simulink model "ScriptDemo"  (R2022b)
settings: configuration reference "TmVcThermal_Configuration_sub" (kept outside this file)
undefined symbols (not defined in the file or in its folder): aaaa, bbbb, cTmComprCtrl_D_u8HvacFlowTable_db, cTmComprCtrl_D_u8HvacFlowTable_sw, cTmComprCtrl_n_i16ChillCmpIMax, cTmComprCtrl_n_i16ChillCmpIMin, cTmComprCtrl_n_i16ChillCmpIMin666, cTmComprCtrl_n_i16ChillCmpPMax, cTmComprCtrl_n_i16ChillCmpPMin, cTmComprCtrl_n_i16CmpChillCoolRpmKiMax, cTmComprCtrl_n_i16CmpChillCoolRpmKiMin, cTmComprCtrl_n_i16CmpChillCoolRpmKpMax, cTmComprCtrl_n_i16CmpChillCoolRpmKpMin, cTmComprCtrl_n_i16CmpCoolRpmKiMax, cTmComprCtrl_n_i16CmpCoolRpmKiMin, cTmComprCtrl_n_i16CmpCoolRpmKpMax, cTmComprCtrl_n_i16CmpCoolRpmKpMin, cTmComprCtrl_n_i16SM4CmpHeatKiMax, cTmComprCtrl_n_i16SM4CmpHeatKiMin, cTmComprCtrl_n_i16SM4CmpHeatKpMax, cTmComprCtrl_n_i16SM4CmpHeatKpMin, cTmComprCtrl_n_i16SM5CmpHeatKiMax, cTmComprCtrl_n_i16SM5CmpHeatKiMin, cTmComprCtrl_n_i16SM5CmpHeatKpMax, cTmComprCtrl_n_i16SM5CmpHeatKpMin, cTmComprCtrl_n_i16SM6CmpHeatKiMax, cTmComprCtrl_n_i16SM6CmpHeatKiMin, cTmComprCtrl_n_i16SM6CmpHeatKpMax, cTmComprCtrl_n_i16SM6CmpHeatKpMin, cTmComprCtrl_n_u16CmpMaxSpdFanFltLimt, cTmComprCtrl_n_u16CmpMaxSpdLoSidePFltLimt, cTmComprCtrl_n_u16CmpMaxSpdSensorFltLimt, cTmComprCtrl_n_u16CompMinRpm, cTmComprCtrl_n_u16CompRpmIncThres, cTmComprCtrl_t_u16BattCooltFFPeriod, cTmComprCtrl_t_u16BattCooltPIPeriod, cTmComprCtrl_t_u16CmpCoolFFPeriod, cTmComprCtrl_t_u16CmpCoolPIPeriod, cTmComprCtrl_t_u16CoolCmpChillFFPeriod, cTmComprCtrl_t_u16CoolCmpChillPIPeriod, cTmComprCtrl_t_u16SM4CmpHeatFFPeriod, cTmComprCtrl_t_u16SM4CmpHeatPIPeriod, cTmComprCtrl_t_u16SM5CmpHeatFFPeriod, cTmComprCtrl_t_u16SM5CmpHeatPIPeriod, cTmComprCtrl_t_u16SM6CmpHeatFFPeriod, cTmComprCtrl_t_u16SM6CmpHeatPIPeriod, cTmComprCtrl_Te_EvapClearInteg, cTmComprCtrl_Te_i16HpReqTempSaturoffset, cTmComprCtrl_Te_i16SatLpReplaceDiff, cTmComprCtrl_Te_i16SM3BatDiffStartEvapDecOffset, cTmComprCtrl_Te_i16SM3EvapLo, cTmComprCtrl_Te_i16SM3TBatDiffEntEvapDecOffset, cTmComprCtrl_Te_i16SM3TBatDiffEntEvapDecOffsetQuit, cTmComprCtrl_Te_s32ErrCmpChillPIContinueCoolH, cTmComprCtrl_Te_s32ErrCmpChillPIContinueCoolL, cTmComprCtrl_Te_s32ErrCmpPIContinueChillH, cTmComprCtrl_Te_s32ErrCmpPIContinueChillL, cTmComprCtrl_Te_s32ErrCmpPIContinueCoolH, cTmComprCtrl_Te_s32ErrCmpPIContinueCoolL, cTmComprCtrl_Te_s32ErrCmpPIContinueHeatH ... (+398)
libraries: simulink x846, PCMULib x711, simulink_need_slupdate x4
(part 11 of 49)

== system ScriptDemo/Create/createSigOnLine/After ==
  note: createSigOnLine(gcs ,'resoveValue',true)
  sTmRefriVlvCtrl_X_s32CEXVPosReqIn : Inport  OutDataTypeStr=single  OutputFunctionCall=on
  sTmRefriVlvCtrl_X_s32EEXVPosReqIn : Inport  Port=2  OutDataTypeStr=single
  sTmRefriVlvCtrl_X_s32BEXVPosReqIn : Inport  Port=3  OutDataTypeStr=single
  yTmRefriVlvCtrl_B_HpcCexvMovEnableIn : Inport  Port=4  OutDataTypeStr=boolean
  sTmRefriVlvCtrl_Z_u8CEXVInitStateIn : Inport  Port=5  OutDataTypeStr=uint8
  yTmRefriVlvCtrl_B_CexvCalibReqIn : Inport  Port=6  OutDataTypeStr=boolean
  yTmRefriVlvCtrl_B_HpcEexvMovEnableIn : Inport  Port=7  OutDataTypeStr=boolean
  sTmRefriVlvCtrl_Z_u8EEXVInitStateIn : Inport  Port=8  OutDataTypeStr=uint8
  yTmRefriVlvCtrl_B_EexvCalibReqIn : Inport  Port=9  OutDataTypeStr=boolean
  yTmRefriVlvCtrl_B_HpcBexvMovEnableIn : Inport  Port=10  OutDataTypeStr=boolean
  sTmRefriVlvCtrl_Z_u8BEXVInitStateIn : Inport  Port=11  OutDataTypeStr=uint8
  yTmRefriVlvCtrl_B_BexvCalibReqIn : Inport  Port=12  OutDataTypeStr=boolean
  sTmRefriVlvCtrl_X_s32SM3BexvMaxPosIn : Inport  Port=13  OutDataTypeStr=single
  yTmRefriVlvCtrl_B_EvapBattTLimBexvEnaIn : Inport  Port=14  OutDataTypeStr=boolean
  sTmRefriVlvCtrl_D_u8EexvRefriSwitchStIn : Inport  Port=15  OutDataTypeStr=uint8
  sTmRefriVlvCtrl_D_u8CexvRefriSwitchStIn : Inport  Port=16  OutDataTypeStr=uint8
  sTmRefriVlvCtrl_D_u8BexvRefriSwitchStIn : Inport  Port=17  OutDataTypeStr=uint8
  Before : Subsystem
  sTmRefriVlvCtrl_X_s32CEXVPosReq : Outport  OutDataTypeStr=single
  sTmRefriVlvCtrl_X_s32EEXVPosReq : Outport  Port=2  OutDataTypeStr=single
  sTmRefriVlvCtrl_X_s32BEXVPosReq : Outport  Port=3  OutDataTypeStr=single
  yTmRefriVlvCtrl_B_HpcCexvMovEnable : Outport  Port=4  OutDataTypeStr=boolean
  sTmRefriVlvCtrl_Z_u8CEXVInitState : Outport  Port=5  OutDataTypeStr=uint8
  yTmRefriVlvCtrl_B_CexvCalibReq : Outport  Port=6  OutDataTypeStr=boolean
  yTmRefriVlvCtrl_B_HpcEexvMovEnable : Outport  Port=7  OutDataTypeStr=boolean
  sTmRefriVlvCtrl_Z_u8EEXVInitState : Outport  Port=8  OutDataTypeStr=uint8
  yTmRefriVlvCtrl_B_EexvCalibReq : Outport  Port=9  OutDataTypeStr=boolean
  yTmRefriVlvCtrl_B_HpcBexvMovEnable : Outport  Port=10  OutDataTypeStr=boolean
  sTmRefriVlvCtrl_Z_u8BEXVInitState : Outport  Port=11  OutDataTypeStr=uint8
  yTmRefriVlvCtrl_B_BexvCalibReq : Outport  Port=12  OutDataTypeStr=boolean
  sTmRefriVlvCtrl_X_s32SM3BexvMaxPos : Outport  Port=13  OutDataTypeStr=single
  yTmRefriVlvCtrl_B_EvapBattTLimBexvEna : Outport  Port=14  OutDataTypeStr=boolean
  sTmRefriVlvCtrl_D_u8EexvRefriSwitchSt : Outport  Port=15  OutDataTypeStr=uint8
  sTmRefriVlvCtrl_D_u8CexvRefriSwitchSt : Outport  Port=16  OutDataTypeStr=uint8
  sTmRefriVlvCtrl_D_u8BexvRefriSwitchSt : Outport  Port=17  OutDataTypeStr=uint8
  wires:
  Before/17(sTmRefriVlvCtrl_D_u8BexvRefriSwitchSt) -> sTmRefriVlvCtrl_D_u8BexvRefriSwitchSt/1  "sTmRefriVlvCtrl_D_u8BexvRefriSwitchSt"
  Before/3(sTmRefriVlvCtrl_X_s32BEXVPosReq) -> sTmRefriVlvCtrl_X_s32BEXVPosReq/1  "sTmRefriVlvCtrl_X_s32BEXVPosReq"
  Before/11(sTmRefriVlvCtrl_Z_u8BEXVInitState) -> sTmRefriVlvCtrl_Z_u8BEXVInitState/1  "sTmRefriVlvCtrl_Z_u8BEXVInitState"
  Before/10(yTmRefriVlvCtrl_B_HpcBexvMovEnable) -> yTmRefriVlvCtrl_B_HpcBexvMovEnable/1  "yTmRefriVlvCtrl_B_HpcBexvMovEnable"
  Before/15(sTmRefriVlvCtrl_D_u8EexvRefriSwitchSt) -> sTmRefriVlvCtrl_D_u8EexvRefriSwitchSt/1  "sTmRefriVlvCtrl_D_u8EexvRefriSwitchSt"
  Before/7(yTmRefriVlvCtrl_B_HpcEexvMovEnable) -> yTmRefriVlvCtrl_B_HpcEexvMovEnable/1  "yTmRefriVlvCtrl_B_HpcEexvMovEnable"
  Before/14(yTmRefriVlvCtrl_B_EvapBattTLimBexvEna) -> yTmRefriVlvCtrl_B_EvapBattTLimBexvEna/1  "yTmRefriVlvCtrl_B_EvapBattTLimBexvEna"
  Before/12(yTmRefriVlvCtrl_B_BexvCalibReq) -> yTmRefriVlvCtrl_B_BexvCalibReq/1  "yTmRefriVlvCtrl_B_BexvCalibReq"
  Before/9(yTmRefriVlvCtrl_B_EexvCalibReq) -> yTmRefriVlvCtrl_B_EexvCalibReq/1  "yTmRefriVlvCtrl_B_EexvCalibReq"
  Before/5(sTmRefriVlvCtrl_Z_u8CEXVInitState) -> sTmRefriVlvCtrl_Z_u8CEXVInitState/1  "sTmRefriVlvCtrl_Z_u8CEXVInitState"
  Before/13(sTmRefriVlvCtrl_X_s32SM3BexvMaxPos) -> sTmRefriVlvCtrl_X_s32SM3BexvMaxPos/1  "sTmRefriVlvCtrl_X_s32SM3BexvMaxPos"
  Before/4(yTmRefriVlvCtrl_B_HpcCexvMovEnable) -> yTmRefriVlvCtrl_B_HpcCexvMovEnable/1  "yTmRefriVlvCtrl_B_HpcCexvMovEnable"
  sTmRefriVlvCtrl_D_u8EexvRefriSwitchStIn/1 -> Before/15(sTmRefriVlvCtrl_D_u8EexvRefriSwitchStIn)  "sTmRefriVlvCtrl_D_u8EexvRefriSwitchStIn"
  yTmRefriVlvCtrl_B_CexvCalibReqIn/1 -> Before/6(yTmRefriVlvCtrl_B_CexvCalibReqIn)  "yTmRefriVlvCtrl_B_CexvCalibReqIn"
  sTmRefriVlvCtrl_D_u8BexvRefriSwitchStIn/1 -> Before/17(sTmRefriVlvCtrl_D_u8BexvRefriSwitchStIn)  "sTmRefriVlvCtrl_D_u8BexvRefriSwitchStIn"
  Before/16(sTmRefriVlvCtrl_D_u8CexvRefriSwitchSt) -> sTmRefriVlvCtrl_D_u8CexvRefriSwitchSt/1  "sTmRefriVlvCtrl_D_u8CexvRefriSwitchSt"
  Before/2(sTmRefriVlvCtrl_X_s32EEXVPosReq) -> sTmRefriVlvCtrl_X_s32EEXVPosReq/1  "sTmRefriVlvCtrl_X_s32EEXVPosReq"
  sTmRefriVlvCtrl_D_u8CexvRefriSwitchStIn/1 -> Before/16(sTmRefriVlvCtrl_D_u8CexvRefriSwitchStIn)  "sTmRefriVlvCtrl_D_u8CexvRefriSwitchStIn"
  yTmRefriVlvCtrl_B_HpcCexvMovEnableIn/1 -> Before/4(yTmRefriVlvCtrl_B_HpcCexvMovEnableIn)  "yTmRefriVlvCtrl_B_HpcCexvMovEnableIn"
  yTmRefriVlvCtrl_B_BexvCalibReqIn/1 -> Before/12(yTmRefriVlvCtrl_B_BexvCalibReqIn)  "yTmRefriVlvCtrl_B_BexvCalibReqIn"
  Before/6(yTmRefriVlvCtrl_B_CexvCalibReq) -> yTmRefriVlvCtrl_B_CexvCalibReq/1  "yTmRefriVlvCtrl_B_CexvCalibReq"
  sTmRefriVlvCtrl_X_s32SM3BexvMaxPosIn/1 -> Before/13(sTmRefriVlvCtrl_X_s32SM3BexvMaxPosIn)  "sTmRefriVlvCtrl_X_s32SM3BexvMaxPosIn"
  yTmRefriVlvCtrl_B_HpcEexvMovEnableIn/1 -> Before/7(yTmRefriVlvCtrl_B_HpcEexvMovEnableIn)  "yTmRefriVlvCtrl_B_HpcEexvMovEnableIn"
  yTmRefriVlvCtrl_B_EexvCalibReqIn/1 -> Before/9(yTmRefriVlvCtrl_B_EexvCalibReqIn)  "yTmRefriVlvCtrl_B_EexvCalibReqIn"
  sTmRefriVlvCtrl_Z_u8CEXVInitStateIn/1 -> Before/5(sTmRefriVlvCtrl_Z_u8CEXVInitStateIn)  "sTmRefriVlvCtrl_Z_u8CEXVInitStateIn"
  sTmRefriVlvCtrl_Z_u8BEXVInitStateIn/1 -> Before/11(sTmRefriVlvCtrl_Z_u8BEXVInitStateIn)  "sTmRefriVlvCtrl_Z_u8BEXVInitStateIn"
  sTmRefriVlvCtrl_X_s32BEXVPosReqIn/1 -> Before/3(sTmRefriVlvCtrl_X_s32BEXVPosReqIn)  "sTmRefriVlvCtrl_X_s32BEXVPosReqIn"
  Before/1(sTmRefriVlvCtrl_X_s32CEXVPosReq) -> sTmRefriVlvCtrl_X_s32CEXVPosReq/1  "sTmRefriVlvCtrl_X_s32CEXVPosReq"
  yTmRefriVlvCtrl_B_HpcBexvMovEnableIn/1 -> Before/10(yTmRefriVlvCtrl_B_HpcBexvMovEnableIn)  "yTmRefriVlvCtrl_B_HpcBexvMovEnableIn"
  sTmRefriVlvCtrl_X_s32EEXVPosReqIn/1 -> Before/2(sTmRefriVlvCtrl_X_s32EEXVPosReqIn)  "sTmRefriVlvCtrl_X_s32EEXVPosReqIn"
  sTmRefriVlvCtrl_Z_u8EEXVInitStateIn/1 -> Before/8(sTmRefriVlvCtrl_Z_u8EEXVInitStateIn)  "sTmRefriVlvCtrl_Z_u8EEXVInitStateIn"
  Before/8(sTmRefriVlvCtrl_Z_u8EEXVInitState) -> sTmRefriVlvCtrl_Z_u8EEXVInitState/1  "sTmRefriVlvCtrl_Z_u8EEXVInitState"
  sTmRefriVlvCtrl_X_s32CEXVPosReqIn/1 -> Before/1(sTmRefriVlvCtrl_X_s32CEXVPosReqIn)  "sTmRefriVlvCtrl_X_s32CEXVPosReqIn"
  yTmRefriVlvCtrl_B_EvapBattTLimBexvEnaIn/1 -> Before/14(yTmRefriVlvCtrl_B_EvapBattTLimBexvEnaIn)  "yTmRefriVlvCtrl_B_EvapBattTLimBexvEnaIn"

== system ScriptDemo/Create/createSigOnLine/After2 ==
  note: createSigOnLine(gcs ,'logValue',true)
  sTmRefriVlvCtrl_X_s32CEXVPosReqIn : Inport  OutDataTypeStr=single  OutputFunctionCall=on
  sTmRefriVlvCtrl_X_s32EEXVPosReqIn : Inport  Port=2  OutDataTypeStr=single
  sTmRefriVlvCtrl_X_s32BEXVPosReqIn : Inport  Port=3  OutDataTypeStr=single
  yTmRefriVlvCtrl_B_HpcCexvMovEnableIn : Inport  Port=4  OutDataTypeStr=boolean
  sTmRefriVlvCtrl_Z_u8CEXVInitStateIn : Inport  Port=5  OutDataTypeStr=uint8
  yTmRefriVlvCtrl_B_CexvCalibReqIn : Inport  Port=6  OutDataTypeStr=boolean
  yTmRefriVlvCtrl_B_HpcEexvMovEnableIn : Inport  Port=7  OutDataTypeStr=boolean
  sTmRefriVlvCtrl_Z_u8EEXVInitStateIn : Inport  Port=8  OutDataTypeStr=uint8
  yTmRefriVlvCtrl_B_EexvCalibReqIn : Inport  Port=9  OutDataTypeStr=boolean
  yTmRefriVlvCtrl_B_HpcBexvMovEnableIn : Inport  Port=10  OutDataTypeStr=boolean
  sTmRefriVlvCtrl_Z_u8BEXVInitStateIn : Inport  Port=11  OutDataTypeStr=uint8
  yTmRefriVlvCtrl_B_BexvCalibReqIn : Inport  Port=12  OutDataTypeStr=boolean
  sTmRefriVlvCtrl_X_s32SM3BexvMaxPosIn : Inport  Port=13  OutDataTypeStr=single
  yTmRefriVlvCtrl_B_EvapBattTLimBexvEnaIn : Inport  Port=14  OutDataTypeStr=boolean
  sTmRefriVlvCtrl_D_u8EexvRefriSwitchStIn : Inport  Port=15  OutDataTypeStr=uint8
  sTmRefriVlvCtrl_D_u8CexvRefriSwitchStIn : Inport  Port=16  OutDataTypeStr=uint8
  sTmRefriVlvCtrl_D_u8BexvRefriSwitchStIn : Inport  Port=17  OutDataTypeStr=uint8
  Before : Subsystem
  sTmRefriVlvCtrl_X_s32CEXVPosReq : Outport  OutDataTypeStr=single
  sTmRefriVlvCtrl_X_s32EEXVPosReq : Outport  Port=2  OutDataTypeStr=single
  sTmRefriVlvCtrl_X_s32BEXVPosReq : Outport  Port=3  OutDataTypeStr=single
  yTmRefriVlvCtrl_B_HpcCexvMovEnable : Outport  Port=4  OutDataTypeStr=boolean
  sTmRefriVlvCtrl_Z_u8CEXVInitState : Outport  Port=5  OutDataTypeStr=uint8
  yTmRefriVlvCtrl_B_CexvCalibReq : Outport  Port=6  OutDataTypeStr=boolean
  yTmRefriVlvCtrl_B_HpcEexvMovEnable : Outport  Port=7  OutDataTypeStr=boolean
  sTmRefriVlvCtrl_Z_u8EEXVInitState : Outport  Port=8  OutDataTypeStr=uint8
  yTmRefriVlvCtrl_B_EexvCalibReq : Outport  Port=9  OutDataTypeStr=boolean
  yTmRefriVlvCtrl_B_HpcBexvMovEnable : Outport  Port=10  OutDataTypeStr=boolean
  sTmRefriVlvCtrl_Z_u8BEXVInitState : Outport  Port=11  OutDataTypeStr=uint8
  yTmRefriVlvCtrl_B_BexvCalibReq : Outport  Port=12  OutDataTypeStr=boolean
  sTmRefriVlvCtrl_X_s32SM3BexvMaxPos : Outport  Port=13  OutDataTypeStr=single
  yTmRefriVlvCtrl_B_EvapBattTLimBexvEna : Outport  Port=14  OutDataTypeStr=boolean
  sTmRefriVlvCtrl_D_u8EexvRefriSwitchSt : Outport  Port=15  OutDataTypeStr=uint8
  sTmRefriVlvCtrl_D_u8CexvRefriSwitchSt : Outport  Port=16  OutDataTypeStr=uint8
  sTmRefriVlvCtrl_D_u8BexvRefriSwitchSt : Outport  Port=17  OutDataTypeStr=uint8
  wires:
  Before/17(sTmRefriVlvCtrl_D_u8BexvRefriSwitchSt) -> sTmRefriVlvCtrl_D_u8BexvRefriSwitchSt/1  "sTmRefriVlvCtrl_D_u8BexvRefriSwitchSt"
  Before/3(sTmRefriVlvCtrl_X_s32BEXVPosReq) -> sTmRefriVlvCtrl_X_s32BEXVPosReq/1  "sTmRefriVlvCtrl_X_s32BEXVPosReq"
  Before/11(sTmRefriVlvCtrl_Z_u8BEXVInitState) -> sTmRefriVlvCtrl_Z_u8BEXVInitState/1  "sTmRefriVlvCtrl_Z_u8BEXVInitState"
  Before/10(yTmRefriVlvCtrl_B_HpcBexvMovEnable) -> yTmRefriVlvCtrl_B_HpcBexvMovEnable/1  "yTmRefriVlvCtrl_B_HpcBexvMovEnable"
  Before/15(sTmRefriVlvCtrl_D_u8EexvRefriSwitchSt) -> sTmRefriVlvCtrl_D_u8EexvRefriSwitchSt/1  "sTmRefriVlvCtrl_D_u8EexvRefriSwitchSt"
  Before/7(yTmRefriVlvCtrl_B_HpcEexvMovEnable) -> yTmRefriVlvCtrl_B_HpcEexvMovEnable/1  "yTmRefriVlvCtrl_B_HpcEexvMovEnable"
  Before/14(yTmRefriVlvCtrl_B_EvapBattTLimBexvEna) -> yTmRefriVlvCtrl_B_EvapBattTLimBexvEna/1  "yTmRefriVlvCtrl_B_EvapBattTLimBexvEna"
  Before/12(yTmRefriVlvCtrl_B_BexvCalibReq) -> yTmRefriVlvCtrl_B_BexvCalibReq/1  "yTmRefriVlvCtrl_B_BexvCalibReq"
  Before/9(yTmRefriVlvCtrl_B_EexvCalibReq) -> yTmRefriVlvCtrl_B_EexvCalibReq/1  "yTmRefriVlvCtrl_B_EexvCalibReq"
  Before/5(sTmRefriVlvCtrl_Z_u8CEXVInitState) -> sTmRefriVlvCtrl_Z_u8CEXVInitState/1  "sTmRefriVlvCtrl_Z_u8CEXVInitState"
  Before/13(sTmRefriVlvCtrl_X_s32SM3BexvMaxPos) -> sTmRefriVlvCtrl_X_s32SM3BexvMaxPos/1  "sTmRefriVlvCtrl_X_s32SM3BexvMaxPos"
  Before/4(yTmRefriVlvCtrl_B_HpcCexvMovEnable) -> yTmRefriVlvCtrl_B_HpcCexvMovEnable/1  "yTmRefriVlvCtrl_B_HpcCexvMovEnable"
  sTmRefriVlvCtrl_D_u8EexvRefriSwitchStIn/1 -> Before/15(sTmRefriVlvCtrl_D_u8EexvRefriSwitchStIn)  "sTmRefriVlvCtrl_D_u8EexvRefriSwitchStIn"
  yTmRefriVlvCtrl_B_CexvCalibReqIn/1 -> Before/6(yTmRefriVlvCtrl_B_CexvCalibReqIn)  "yTmRefriVlvCtrl_B_CexvCalibReqIn"
  sTmRefriVlvCtrl_D_u8BexvRefriSwitchStIn/1 -> Before/17(sTmRefriVlvCtrl_D_u8BexvRefriSwitchStIn)  "sTmRefriVlvCtrl_D_u8BexvRefriSwitchStIn"
  Before/16(sTmRefriVlvCtrl_D_u8CexvRefriSwitchSt) -> sTmRefriVlvCtrl_D_u8CexvRefriSwitchSt/1  "sTmRefriVlvCtrl_D_u8CexvRefriSwitchSt"
  Before/2(sTmRefriVlvCtrl_X_s32EEXVPosReq) -> sTmRefriVlvCtrl_X_s32EEXVPosReq/1  "sTmRefriVlvCtrl_X_s32EEXVPosReq"
  sTmRefriVlvCtrl_D_u8CexvRefriSwitchStIn/1 -> Before/16(sTmRefriVlvCtrl_D_u8CexvRefriSwitchStIn)  "sTmRefriVlvCtrl_D_u8CexvRefriSwitchStIn"
  yTmRefriVlvCtrl_B_HpcCexvMovEnableIn/1 -> Before/4(yTmRefriVlvCtrl_B_HpcCexvMovEnableIn)  "yTmRefriVlvCtrl_B_HpcCexvMovEnableIn"
  yTmRefriVlvCtrl_B_BexvCalibReqIn/1 -> Before/12(yTmRefriVlvCtrl_B_BexvCalibReqIn)  "yTmRefriVlvCtrl_B_BexvCalibReqIn"
  Before/6(yTmRefriVlvCtrl_B_CexvCalibReq) -> yTmRefriVlvCtrl_B_CexvCalibReq/1  "yTmRefriVlvCtrl_B_CexvCalibReq"
  sTmRefriVlvCtrl_X_s32SM3BexvMaxPosIn/1 -> Before/13(sTmRefriVlvCtrl_X_s32SM3BexvMaxPosIn)  "sTmRefriVlvCtrl_X_s32SM3BexvMaxPosIn"
  yTmRefriVlvCtrl_B_HpcEexvMovEnableIn/1 -> Before/7(yTmRefriVlvCtrl_B_HpcEexvMovEnableIn)  "yTmRefriVlvCtrl_B_HpcEexvMovEnableIn"
  yTmRefriVlvCtrl_B_EexvCalibReqIn/1 -> Before/9(yTmRefriVlvCtrl_B_EexvCalibReqIn)  "yTmRefriVlvCtrl_B_EexvCalibReqIn"
  sTmRefriVlvCtrl_Z_u8CEXVInitStateIn/1 -> Before/5(sTmRefriVlvCtrl_Z_u8CEXVInitStateIn)  "sTmRefriVlvCtrl_Z_u8CEXVInitStateIn"
  sTmRefriVlvCtrl_Z_u8BEXVInitStateIn/1 -> Before/11(sTmRefriVlvCtrl_Z_u8BEXVInitStateIn)  "sTmRefriVlvCtrl_Z_u8BEXVInitStateIn"
  sTmRefriVlvCtrl_X_s32BEXVPosReqIn/1 -> Before/3(sTmRefriVlvCtrl_X_s32BEXVPosReqIn)  "sTmRefriVlvCtrl_X_s32BEXVPosReqIn"
  Before/1(sTmRefriVlvCtrl_X_s32CEXVPosReq) -> sTmRefriVlvCtrl_X_s32CEXVPosReq/1  "sTmRefriVlvCtrl_X_s32CEXVPosReq"
  yTmRefriVlvCtrl_B_HpcBexvMovEnableIn/1 -> Before/10(yTmRefriVlvCtrl_B_HpcBexvMovEnableIn)  "yTmRefriVlvCtrl_B_HpcBexvMovEnableIn"
  sTmRefriVlvCtrl_X_s32EEXVPosReqIn/1 -> Before/2(sTmRefriVlvCtrl_X_s32EEXVPosReqIn)  "sTmRefriVlvCtrl_X_s32EEXVPosReqIn"
  sTmRefriVlvCtrl_Z_u8EEXVInitStateIn/1 -> Before/8(sTmRefriVlvCtrl_Z_u8EEXVInitStateIn)  "sTmRefriVlvCtrl_Z_u8EEXVInitStateIn"
  Before/8(sTmRefriVlvCtrl_Z_u8EEXVInitState) -> sTmRefriVlvCtrl_Z_u8EEXVInitState/1  "sTmRefriVlvCtrl_Z_u8EEXVInitState"
  sTmRefriVlvCtrl_X_s32CEXVPosReqIn/1 -> Before/1(sTmRefriVlvCtrl_X_s32CEXVPosReqIn)  "sTmRefriVlvCtrl_X_s32CEXVPosReqIn"
  yTmRefriVlvCtrl_B_EvapBattTLimBexvEnaIn/1 -> Before/14(yTmRefriVlvCtrl_B_EvapBattTLimBexvEnaIn)  "yTmRefriVlvCtrl_B_EvapBattTLimBexvEnaIn"

== system ScriptDemo/Create/createSigOnLine/After3 ==
  note: createSigOnLine(gcs ,' testValue ',true)
  sTmRefriVlvCtrl_X_s32CEXVPosReqIn : Inport  OutDataTypeStr=single  OutputFunctionCall=on
  sTmRefriVlvCtrl_X_s32EEXVPosReqIn : Inport  Port=2  OutDataTypeStr=single
  sTmRefriVlvCtrl_X_s32BEXVPosReqIn : Inport  Port=3  OutDataTypeStr=single
  yTmRefriVlvCtrl_B_HpcCexvMovEnableIn : Inport  Port=4  OutDataTypeStr=boolean
  sTmRefriVlvCtrl_Z_u8CEXVInitStateIn : Inport  Port=5  OutDataTypeStr=uint8
  yTmRefriVlvCtrl_B_CexvCalibReqIn : Inport  Port=6  OutDataTypeStr=boolean
  yTmRefriVlvCtrl_B_HpcEexvMovEnableIn : Inport  Port=7  OutDataTypeStr=boolean
  sTmRefriVlvCtrl_Z_u8EEXVInitStateIn : Inport  Port=8  OutDataTypeStr=uint8
  yTmRefriVlvCtrl_B_EexvCalibReqIn : Inport  Port=9  OutDataTypeStr=boolean
  yTmRefriVlvCtrl_B_HpcBexvMovEnableIn : Inport  Port=10  OutDataTypeStr=boolean
  sTmRefriVlvCtrl_Z_u8BEXVInitStateIn : Inport  Port=11  OutDataTypeStr=uint8
  yTmRefriVlvCtrl_B_BexvCalibReqIn : Inport  Port=12  OutDataTypeStr=boolean
  sTmRefriVlvCtrl_X_s32SM3BexvMaxPosIn : Inport  Port=13  OutDataTypeStr=single
  yTmRefriVlvCtrl_B_EvapBattTLimBexvEnaIn : Inport  Port=14  OutDataTypeStr=boolean
  sTmRefriVlvCtrl_D_u8EexvRefriSwitchStIn : Inport  Port=15  OutDataTypeStr=uint8
  sTmRefriVlvCtrl_D_u8CexvRefriSwitchStIn : Inport  Port=16  OutDataTypeStr=uint8
  sTmRefriVlvCtrl_D_u8BexvRefriSwitchStIn : Inport  Port=17  OutDataTypeStr=uint8
  Before : Subsystem
  sTmRefriVlvCtrl_X_s32CEXVPosReq : Outport  OutDataTypeStr=single
  sTmRefriVlvCtrl_X_s32EEXVPosReq : Outport  Port=2  OutDataTypeStr=single
  sTmRefriVlvCtrl_X_s32BEXVPosReq : Outport  Port=3  OutDataTypeStr=single
  yTmRefriVlvCtrl_B_HpcCexvMovEnable : Outport  Port=4  OutDataTypeStr=boolean
  sTmRefriVlvCtrl_Z_u8CEXVInitState : Outport  Port=5  OutDataTypeStr=uint8
  yTmRefriVlvCtrl_B_CexvCalibReq : Outport  Port=6  OutDataTypeStr=boolean
  yTmRefriVlvCtrl_B_HpcEexvMovEnable : Outport  Port=7  OutDataTypeStr=boolean
  sTmRefriVlvCtrl_Z_u8EEXVInitState : Outport  Port=8  OutDataTypeStr=uint8
  yTmRefriVlvCtrl_B_EexvCalibReq : Outport  Port=9  OutDataTypeStr=boolean
  yTmRefriVlvCtrl_B_HpcBexvMovEnable : Outport  Port=10  OutDataTypeStr=boolean
  sTmRefriVlvCtrl_Z_u8BEXVInitState : Outport  Port=11  OutDataTypeStr=uint8
  yTmRefriVlvCtrl_B_BexvCalibReq : Outport  Port=12  OutDataTypeStr=boolean
  sTmRefriVlvCtrl_X_s32SM3BexvMaxPos : Outport  Port=13  OutDataTypeStr=single
  yTmRefriVlvCtrl_B_EvapBattTLimBexvEna : Outport  Port=14  OutDataTypeStr=boolean
  sTmRefriVlvCtrl_D_u8EexvRefriSwitchSt : Outport  Port=15  OutDataTypeStr=uint8
  sTmRefriVlvCtrl_D_u8CexvRefriSwitchSt : Outport  Port=16  OutDataTypeStr=uint8
  sTmRefriVlvCtrl_D_u8BexvRefriSwitchSt : Outport  Port=17  OutDataTypeStr=uint8
  wires:
  Before/17(sTmRefriVlvCtrl_D_u8BexvRefriSwitchSt) -> sTmRefriVlvCtrl_D_u8BexvRefriSwitchSt/1  "sTmRefriVlvCtrl_D_u8BexvRefriSwitchSt"
  Before/3(sTmRefriVlvCtrl_X_s32BEXVPosReq) -> sTmRefriVlvCtrl_X_s32BEXVPosReq/1  "sTmRefriVlvCtrl_X_s32BEXVPosReq"
  Before/11(sTmRefriVlvCtrl_Z_u8BEXVInitState) -> sTmRefriVlvCtrl_Z_u8BEXVInitState/1  "sTmRefriVlvCtrl_Z_u8BEXVInitState"
  Before/10(yTmRefriVlvCtrl_B_HpcBexvMovEnable) -> yTmRefriVlvCtrl_B_HpcBexvMovEnable/1  "yTmRefriVlvCtrl_B_HpcBexvMovEnable"
  Before/15(sTmRefriVlvCtrl_D_u8EexvRefriSwitchSt) -> sTmRefriVlvCtrl_D_u8EexvRefriSwitchSt/1  "sTmRefriVlvCtrl_D_u8EexvRefriSwitchSt"
  Before/7(yTmRefriVlvCtrl_B_HpcEexvMovEnable) -> yTmRefriVlvCtrl_B_HpcEexvMovEnable/1  "yTmRefriVlvCtrl_B_HpcEexvMovEnable"
  Before/14(yTmRefriVlvCtrl_B_EvapBattTLimBexvEna) -> yTmRefriVlvCtrl_B_EvapBattTLimBexvEna/1  "yTmRefriVlvCtrl_B_EvapBattTLimBexvEna"
  Before/12(yTmRefriVlvCtrl_B_BexvCalibReq) -> yTmRefriVlvCtrl_B_BexvCalibReq/1  "yTmRefriVlvCtrl_B_BexvCalibReq"
  Before/9(yTmRefriVlvCtrl_B_EexvCalibReq) -> yTmRefriVlvCtrl_B_EexvCalibReq/1  "yTmRefriVlvCtrl_B_EexvCalibReq"
  Before/5(sTmRefriVlvCtrl_Z_u8CEXVInitState) -> sTmRefriVlvCtrl_Z_u8CEXVInitState/1  "sTmRefriVlvCtrl_Z_u8CEXVInitState"
  Before/13(sTmRefriVlvCtrl_X_s32SM3BexvMaxPos) -> sTmRefriVlvCtrl_X_s32SM3BexvMaxPos/1  "sTmRefriVlvCtrl_X_s32SM3BexvMaxPos"
  Before/4(yTmRefriVlvCtrl_B_HpcCexvMovEnable) -> yTmRefriVlvCtrl_B_HpcCexvMovEnable/1  "yTmRefriVlvCtrl_B_HpcCexvMovEnable"
  sTmRefriVlvCtrl_D_u8EexvRefriSwitchStIn/1 -> Before/15(sTmRefriVlvCtrl_D_u8EexvRefriSwitchStIn)  "sTmRefriVlvCtrl_D_u8EexvRefriSwitchStIn"
  yTmRefriVlvCtrl_B_CexvCalibReqIn/1 -> Before/6(yTmRefriVlvCtrl_B_CexvCalibReqIn)  "yTmRefriVlvCtrl_B_CexvCalibReqIn"
  sTmRefriVlvCtrl_D_u8BexvRefriSwitchStIn/1 -> Before/17(sTmRefriVlvCtrl_D_u8BexvRefriSwitchStIn)  "sTmRefriVlvCtrl_D_u8BexvRefriSwitchStIn"
  Before/16(sTmRefriVlvCtrl_D_u8CexvRefriSwitchSt) -> sTmRefriVlvCtrl_D_u8CexvRefriSwitchSt/1  "sTmRefriVlvCtrl_D_u8CexvRefriSwitchSt"
  Before/2(sTmRefriVlvCtrl_X_s32EEXVPosReq) -> sTmRefriVlvCtrl_X_s32EEXVPosReq/1  "sTmRefriVlvCtrl_X_s32EEXVPosReq"
  sTmRefriVlvCtrl_D_u8CexvRefriSwitchStIn/1 -> Before/16(sTmRefriVlvCtrl_D_u8CexvRefriSwitchStIn)  "sTmRefriVlvCtrl_D_u8CexvRefriSwitchStIn"
  yTmRefriVlvCtrl_B_HpcCexvMovEnableIn/1 -> Before/4(yTmRefriVlvCtrl_B_HpcCexvMovEnableIn)  "yTmRefriVlvCtrl_B_HpcCexvMovEnableIn"
  yTmRefriVlvCtrl_B_BexvCalibReqIn/1 -> Before/12(yTmRefriVlvCtrl_B_BexvCalibReqIn)  "yTmRefriVlvCtrl_B_BexvCalibReqIn"
  Before/6(yTmRefriVlvCtrl_B_CexvCalibReq) -> yTmRefriVlvCtrl_B_CexvCalibReq/1  "yTmRefriVlvCtrl_B_CexvCalibReq"
  sTmRefriVlvCtrl_X_s32SM3BexvMaxPosIn/1 -> Before/13(sTmRefriVlvCtrl_X_s32SM3BexvMaxPosIn)  "sTmRefriVlvCtrl_X_s32SM3BexvMaxPosIn"
  yTmRefriVlvCtrl_B_HpcEexvMovEnableIn/1 -> Before/7(yTmRefriVlvCtrl_B_HpcEexvMovEnableIn)  "yTmRefriVlvCtrl_B_HpcEexvMovEnableIn"
  yTmRefriVlvCtrl_B_EexvCalibReqIn/1 -> Before/9(yTmRefriVlvCtrl_B_EexvCalibReqIn)  "yTmRefriVlvCtrl_B_EexvCalibReqIn"
  sTmRefriVlvCtrl_Z_u8CEXVInitStateIn/1 -> Before/5(sTmRefriVlvCtrl_Z_u8CEXVInitStateIn)  "sTmRefriVlvCtrl_Z_u8CEXVInitStateIn"
  sTmRefriVlvCtrl_Z_u8BEXVInitStateIn/1 -> Before/11(sTmRefriVlvCtrl_Z_u8BEXVInitStateIn)  "sTmRefriVlvCtrl_Z_u8BEXVInitStateIn"
  sTmRefriVlvCtrl_X_s32BEXVPosReqIn/1 -> Before/3(sTmRefriVlvCtrl_X_s32BEXVPosReqIn)  "sTmRefriVlvCtrl_X_s32BEXVPosReqIn"
  Before/1(sTmRefriVlvCtrl_X_s32CEXVPosReq) -> sTmRefriVlvCtrl_X_s32CEXVPosReq/1  "sTmRefriVlvCtrl_X_s32CEXVPosReq"
  yTmRefriVlvCtrl_B_HpcBexvMovEnableIn/1 -> Before/10(yTmRefriVlvCtrl_B_HpcBexvMovEnableIn)  "yTmRefriVlvCtrl_B_HpcBexvMovEnableIn"
  sTmRefriVlvCtrl_X_s32EEXVPosReqIn/1 -> Before/2(sTmRefriVlvCtrl_X_s32EEXVPosReqIn)  "sTmRefriVlvCtrl_X_s32EEXVPosReqIn"
  sTmRefriVlvCtrl_Z_u8EEXVInitStateIn/1 -> Before/8(sTmRefriVlvCtrl_Z_u8EEXVInitStateIn)  "sTmRefriVlvCtrl_Z_u8EEXVInitStateIn"
  Before/8(sTmRefriVlvCtrl_Z_u8EEXVInitState) -> sTmRefriVlvCtrl_Z_u8EEXVInitState/1  "sTmRefriVlvCtrl_Z_u8EEXVInitState"
  sTmRefriVlvCtrl_X_s32CEXVPosReqIn/1 -> Before/1(sTmRefriVlvCtrl_X_s32CEXVPosReqIn)  "sTmRefriVlvCtrl_X_s32CEXVPosReqIn"
  yTmRefriVlvCtrl_B_EvapBattTLimBexvEnaIn/1 -> Before/14(yTmRefriVlvCtrl_B_EvapBattTLimBexvEnaIn)  "yTmRefriVlvCtrl_B_EvapBattTLimBexvEnaIn"

== system ScriptDemo/Create/createSigOnLine/After4 ==
  note: createSigOnLine(gcs ,' resoveValue ',true, 'isEnableIn' ,true, 'isEnableOut' ,false )
  sTmRefriVlvCtrl_X_s32CEXVPosReqIn : Inport  OutDataTypeStr=single  OutputFunctionCall=on
  sTmRefriVlvCtrl_X_s32EEXVPosReqIn : Inport  Port=2  OutDataTypeStr=single
  sTmRefriVlvCtrl_X_s32BEXVPosReqIn : Inport  Port=3  OutDataTypeStr=single
  yTmRefriVlvCtrl_B_HpcCexvMovEnableIn : Inport  Port=4  OutDataTypeStr=boolean
  sTmRefriVlvCtrl_Z_u8CEXVInitStateIn : Inport  Port=5  OutDataTypeStr=uint8
  yTmRefriVlvCtrl_B_CexvCalibReqIn : Inport  Port=6  OutDataTypeStr=boolean
  yTmRefriVlvCtrl_B_HpcEexvMovEnableIn : Inport  Port=7  OutDataTypeStr=boolean
  sTmRefriVlvCtrl_Z_u8EEXVInitStateIn : Inport  Port=8  OutDataTypeStr=uint8
  yTmRefriVlvCtrl_B_EexvCalibReqIn : Inport  Port=9  OutDataTypeStr=boolean
  yTmRefriVlvCtrl_B_HpcBexvMovEnableIn : Inport  Port=10  OutDataTypeStr=boolean
  sTmRefriVlvCtrl_Z_u8BEXVInitStateIn : Inport  Port=11  OutDataTypeStr=uint8
  yTmRefriVlvCtrl_B_BexvCalibReqIn : Inport  Port=12  OutDataTypeStr=boolean
  sTmRefriVlvCtrl_X_s32SM3BexvMaxPosIn : Inport  Port=13  OutDataTypeStr=single
  yTmRefriVlvCtrl_B_EvapBattTLimBexvEnaIn : Inport  Port=14  OutDataTypeStr=boolean
  sTmRefriVlvCtrl_D_u8EexvRefriSwitchStIn : Inport  Port=15  OutDataTypeStr=uint8
  sTmRefriVlvCtrl_D_u8CexvRefriSwitchStIn : Inport  Port=16  OutDataTypeStr=uint8
  sTmRefriVlvCtrl_D_u8BexvRefriSwitchStIn : Inport  Port=17  OutDataTypeStr=uint8
  Before : Subsystem
  sTmRefriVlvCtrl_X_s32CEXVPosReq : Outport  OutDataTypeStr=single
  sTmRefriVlvCtrl_X_s32EEXVPosReq : Outport  Port=2  OutDataTypeStr=single
  sTmRefriVlvCtrl_X_s32BEXVPosReq : Outport  Port=3  OutDataTypeStr=single
  yTmRefriVlvCtrl_B_HpcCexvMovEnable : Outport  Port=4  OutDataTypeStr=boolean
  sTmRefriVlvCtrl_Z_u8CEXVInitState : Outport  Port=5  OutDataTypeStr=uint8
  yTmRefriVlvCtrl_B_CexvCalibReq : Outport  Port=6  OutDataTypeStr=boolean
  yTmRefriVlvCtrl_B_HpcEexvMovEnable : Outport  Port=7  OutDataTypeStr=boolean
  sTmRefriVlvCtrl_Z_u8EEXVInitState : Outport  Port=8  OutDataTypeStr=uint8
  yTmRefriVlvCtrl_B_EexvCalibReq : Outport  Port=9  OutDataTypeStr=boolean
  yTmRefriVlvCtrl_B_HpcBexvMovEnable : Outport  Port=10  OutDataTypeStr=boolean
  sTmRefriVlvCtrl_Z_u8BEXVInitState : Outport  Port=11  OutDataTypeStr=uint8
  yTmRefriVlvCtrl_B_BexvCalibReq : Outport  Port=12  OutDataTypeStr=boolean
  sTmRefriVlvCtrl_X_s32SM3BexvMaxPos : Outport  Port=13  OutDataTypeStr=single
  yTmRefriVlvCtrl_B_EvapBattTLimBexvEna : Outport  Port=14  OutDataTypeStr=boolean
  sTmRefriVlvCtrl_D_u8EexvRefriSwitchSt : Outport  Port=15  OutDataTypeStr=uint8
  sTmRefriVlvCtrl_D_u8CexvRefriSwitchSt : Outport  Port=16  OutDataTypeStr=uint8
  sTmRefriVlvCtrl_D_u8BexvRefriSwitchSt : Outport  Port=17  OutDataTypeStr=uint8
  wires:
  Before/17(sTmRefriVlvCtrl_D_u8BexvRefriSwitchSt) -> sTmRefriVlvCtrl_D_u8BexvRefriSwitchSt/1
  Before/3(sTmRefriVlvCtrl_X_s32BEXVPosReq) -> sTmRefriVlvCtrl_X_s32BEXVPosReq/1
  Before/11(sTmRefriVlvCtrl_Z_u8BEXVInitState) -> sTmRefriVlvCtrl_Z_u8BEXVInitState/1
  Before/10(yTmRefriVlvCtrl_B_HpcBexvMovEnable) -> yTmRefriVlvCtrl_B_HpcBexvMovEnable/1
  Before/15(sTmRefriVlvCtrl_D_u8EexvRefriSwitchSt) -> sTmRefriVlvCtrl_D_u8EexvRefriSwitchSt/1
  Before/7(yTmRefriVlvCtrl_B_HpcEexvMovEnable) -> yTmRefriVlvCtrl_B_HpcEexvMovEnable/1
  Before/14(yTmRefriVlvCtrl_B_EvapBattTLimBexvEna) -> yTmRefriVlvCtrl_B_EvapBattTLimBexvEna/1
  Before/12(yTmRefriVlvCtrl_B_BexvCalibReq) -> yTmRefriVlvCtrl_B_BexvCalibReq/1
  Before/9(yTmRefriVlvCtrl_B_EexvCalibReq) -> yTmRefriVlvCtrl_B_EexvCalibReq/1
  Before/5(sTmRefriVlvCtrl_Z_u8CEXVInitState) -> sTmRefriVlvCtrl_Z_u8CEXVInitState/1
  Before/13(sTmRefriVlvCtrl_X_s32SM3BexvMaxPos) -> sTmRefriVlvCtrl_X_s32SM3BexvMaxPos/1
  Before/4(yTmRefriVlvCtrl_B_HpcCexvMovEnable) -> yTmRefriVlvCtrl_B_HpcCexvMovEnable/1
  sTmRefriVlvCtrl_D_u8EexvRefriSwitchStIn/1 -> Before/15(sTmRefriVlvCtrl_D_u8EexvRefriSwitchStIn)  "sTmRefriVlvCtrl_D_u8EexvRefriSwitchStIn"
  yTmRefriVlvCtrl_B_CexvCalibReqIn/1 -> Before/6(yTmRefriVlvCtrl_B_CexvCalibReqIn)  "yTmRefriVlvCtrl_B_CexvCalibReqIn"
  sTmRefriVlvCtrl_D_u8BexvRefriSwitchStIn/1 -> Before/17(sTmRefriVlvCtrl_D_u8BexvRefriSwitchStIn)  "sTmRefriVlvCtrl_D_u8BexvRefriSwitchStIn"
  Before/16(sTmRefriVlvCtrl_D_u8CexvRefriSwitchSt) -> sTmRefriVlvCtrl_D_u8CexvRefriSwitchSt/1
  Before/2(sTmRefriVlvCtrl_X_s32EEXVPosReq) -> sTmRefriVlvCtrl_X_s32EEXVPosReq/1
  sTmRefriVlvCtrl_D_u8CexvRefriSwitchStIn/1 -> Before/16(sTmRefriVlvCtrl_D_u8CexvRefriSwitchStIn)  "sTmRefriVlvCtrl_D_u8CexvRefriSwitchStIn"
  yTmRefriVlvCtrl_B_HpcCexvMovEnableIn/1 -> Before/4(yTmRefriVlvCtrl_B_HpcCexvMovEnableIn)  "yTmRefriVlvCtrl_B_HpcCexvMovEnableIn"
  yTmRefriVlvCtrl_B_BexvCalibReqIn/1 -> Before/12(yTmRefriVlvCtrl_B_BexvCalibReqIn)  "yTmRefriVlvCtrl_B_BexvCalibReqIn"
  Before/6(yTmRefriVlvCtrl_B_CexvCalibReq) -> yTmRefriVlvCtrl_B_CexvCalibReq/1
  sTmRefriVlvCtrl_X_s32SM3BexvMaxPosIn/1 -> Before/13(sTmRefriVlvCtrl_X_s32SM3BexvMaxPosIn)  "sTmRefriVlvCtrl_X_s32SM3BexvMaxPosIn"
  yTmRefriVlvCtrl_B_HpcEexvMovEnableIn/1 -> Before/7(yTmRefriVlvCtrl_B_HpcEexvMovEnableIn)  "yTmRefriVlvCtrl_B_HpcEexvMovEnableIn"
  yTmRefriVlvCtrl_B_EexvCalibReqIn/1 -> Before/9(yTmRefriVlvCtrl_B_EexvCalibReqIn)  "yTmRefriVlvCtrl_B_EexvCalibReqIn"
  sTmRefriVlvCtrl_Z_u8CEXVInitStateIn/1 -> Before/5(sTmRefriVlvCtrl_Z_u8CEXVInitStateIn)  "sTmRefriVlvCtrl_Z_u8CEXVInitStateIn"
  sTmRefriVlvCtrl_Z_u8BEXVInitStateIn/1 -> Before/11(sTmRefriVlvCtrl_Z_u8BEXVInitStateIn)  "sTmRefriVlvCtrl_Z_u8BEXVInitStateIn"
  sTmRefriVlvCtrl_X_s32BEXVPosReqIn/1 -> Before/3(sTmRefriVlvCtrl_X_s32BEXVPosReqIn)  "sTmRefriVlvCtrl_X_s32BEXVPosReqIn"
  Before/1(sTmRefriVlvCtrl_X_s32CEXVPosReq) -> sTmRefriVlvCtrl_X_s32CEXVPosReq/1
  yTmRefriVlvCtrl_B_HpcBexvMovEnableIn/1 -> Before/10(yTmRefriVlvCtrl_B_HpcBexvMovEnableIn)  "yTmRefriVlvCtrl_B_HpcBexvMovEnableIn"
  sTmRefriVlvCtrl_X_s32EEXVPosReqIn/1 -> Before/2(sTmRefriVlvCtrl_X_s32EEXVPosReqIn)  "sTmRefriVlvCtrl_X_s32EEXVPosReqIn"
  sTmRefriVlvCtrl_Z_u8EEXVInitStateIn/1 -> Before/8(sTmRefriVlvCtrl_Z_u8EEXVInitStateIn)  "sTmRefriVlvCtrl_Z_u8EEXVInitStateIn"
  Before/8(sTmRefriVlvCtrl_Z_u8EEXVInitState) -> sTmRefriVlvCtrl_Z_u8EEXVInitState/1
  sTmRefriVlvCtrl_X_s32CEXVPosReqIn/1 -> Before/1(sTmRefriVlvCtrl_X_s32CEXVPosReqIn)  "sTmRefriVlvCtrl_X_s32CEXVPosReqIn"
  yTmRefriVlvCtrl_B_EvapBattTLimBexvEnaIn/1 -> Before/14(yTmRefriVlvCtrl_B_EvapBattTLimBexvEnaIn)  "yTmRefriVlvCtrl_B_EvapBattTLimBexvEnaIn"

== system ScriptDemo/Create/createSigOnLine/Before ==
  sTmRefriVlvCtrl_X_s32CEXVPosReqIn : Inport  OutDataTypeStr=single  OutputFunctionCall=on
  sTmRefriVlvCtrl_X_s32EEXVPosReqIn : Inport  Port=2  OutDataTypeStr=single
  sTmRefriVlvCtrl_X_s32BEXVPosReqIn : Inport  Port=3  OutDataTypeStr=single
  yTmRefriVlvCtrl_B_HpcCexvMovEnableIn : Inport  Port=4  OutDataTypeStr=boolean
  sTmRefriVlvCtrl_Z_u8CEXVInitStateIn : Inport  Port=5  OutDataTypeStr=uint8
  yTmRefriVlvCtrl_B_CexvCalibReqIn : Inport  Port=6  OutDataTypeStr=boolean
  yTmRefriVlvCtrl_B_HpcEexvMovEnableIn : Inport  Port=7  OutDataTypeStr=boolean
  sTmRefriVlvCtrl_Z_u8EEXVInitStateIn : Inport  Port=8  OutDataTypeStr=uint8
  yTmRefriVlvCtrl_B_EexvCalibReqIn : Inport  Port=9  OutDataTypeStr=boolean
  yTmRefriVlvCtrl_B_HpcBexvMovEnableIn : Inport  Port=10  OutDataTypeStr=boolean
  sTmRefriVlvCtrl_Z_u8BEXVInitStateIn : Inport  Port=11  OutDataTypeStr=uint8
  yTmRefriVlvCtrl_B_BexvCalibReqIn : Inport  Port=12  OutDataTypeStr=boolean
  sTmRefriVlvCtrl_X_s32SM3BexvMaxPosIn : Inport  Port=13  OutDataTypeStr=single
  yTmRefriVlvCtrl_B_EvapBattTLimBexvEnaIn : Inport  Port=14  OutDataTypeStr=boolean
  sTmRefriVlvCtrl_D_u8EexvRefriSwitchStIn : Inport  Port=15  OutDataTypeStr=uint8
  sTmRefriVlvCtrl_D_u8CexvRefriSwitchStIn : Inport  Port=16  OutDataTypeStr=uint8
  sTmRefriVlvCtrl_D_u8BexvRefriSwitchStIn : Inport  Port=17  OutDataTypeStr=uint8
  Before : Subsystem
  sTmRefriVlvCtrl_X_s32CEXVPosReq : Outport  OutDataTypeStr=single
  sTmRefriVlvCtrl_X_s32EEXVPosReq : Outport  Port=2  OutDataTypeStr=single
  sTmRefriVlvCtrl_X_s32BEXVPosReq : Outport  Port=3  OutDataTypeStr=single
  yTmRefriVlvCtrl_B_HpcCexvMovEnable : Outport  Port=4  OutDataTypeStr=boolean
  sTmRefriVlvCtrl_Z_u8CEXVInitState : Outport  Port=5  OutDataTypeStr=uint8
  yTmRefriVlvCtrl_B_CexvCalibReq : Outport  Port=6  OutDataTypeStr=boolean
  yTmRefriVlvCtrl_B_HpcEexvMovEnable : Outport  Port=7  OutDataTypeStr=boolean
  sTmRefriVlvCtrl_Z_u8EEXVInitState : Outport  Port=8  OutDataTypeStr=uint8
  yTmRefriVlvCtrl_B_EexvCalibReq : Outport  Port=9  OutDataTypeStr=boolean
  yTmRefriVlvCtrl_B_HpcBexvMovEnable : Outport  Port=10  OutDataTypeStr=boolean
  sTmRefriVlvCtrl_Z_u8BEXVInitState : Outport  Port=11  OutDataTypeStr=uint8
  yTmRefriVlvCtrl_B_BexvCalibReq : Outport  Port=12  OutDataTypeStr=boolean
  sTmRefriVlvCtrl_X_s32SM3BexvMaxPos : Outport  Port=13  OutDataTypeStr=single
  yTmRefriVlvCtrl_B_EvapBattTLimBexvEna : Outport  Port=14  OutDataTypeStr=boolean
  sTmRefriVlvCtrl_D_u8EexvRefriSwitchSt : Outport  Port=15  OutDataTypeStr=uint8
  sTmRefriVlvCtrl_D_u8CexvRefriSwitchSt : Outport  Port=16  OutDataTypeStr=uint8
  sTmRefriVlvCtrl_D_u8BexvRefriSwitchSt : Outport  Port=17  OutDataTypeStr=uint8
  wires:
  sTmRefriVlvCtrl_X_s32CEXVPosReqIn/1 -> Before/1(sTmRefriVlvCtrl_X_s32CEXVPosReqIn)
  sTmRefriVlvCtrl_X_s32EEXVPosReqIn/1 -> Before/2(sTmRefriVlvCtrl_X_s32EEXVPosReqIn)
  sTmRefriVlvCtrl_X_s32BEXVPosReqIn/1 -> Before/3(sTmRefriVlvCtrl_X_s32BEXVPosReqIn)
  yTmRefriVlvCtrl_B_HpcCexvMovEnableIn/1 -> Before/4(yTmRefriVlvCtrl_B_HpcCexvMovEnableIn)
  sTmRefriVlvCtrl_Z_u8CEXVInitStateIn/1 -> Before/5(sTmRefriVlvCtrl_Z_u8CEXVInitStateIn)
  yTmRefriVlvCtrl_B_CexvCalibReqIn/1 -> Before/6(yTmRefriVlvCtrl_B_CexvCalibReqIn)
  yTmRefriVlvCtrl_B_HpcEexvMovEnableIn/1 -> Before/7(yTmRefriVlvCtrl_B_HpcEexvMovEnableIn)
  sTmRefriVlvCtrl_Z_u8EEXVInitStateIn/1 -> Before/8(sTmRefriVlvCtrl_Z_u8EEXVInitStateIn)
  yTmRefriVlvCtrl_B_EexvCalibReqIn/1 -> Before/9(yTmRefriVlvCtrl_B_EexvCalibReqIn)
  yTmRefriVlvCtrl_B_HpcBexvMovEnableIn/1 -> Before/10(yTmRefriVlvCtrl_B_HpcBexvMovEnableIn)
  sTmRefriVlvCtrl_Z_u8BEXVInitStateIn/1 -> Before/11(sTmRefriVlvCtrl_Z_u8BEXVInitStateIn)
  yTmRefriVlvCtrl_B_BexvCalibReqIn/1 -> Before/12(yTmRefriVlvCtrl_B_BexvCalibReqIn)
  sTmRefriVlvCtrl_X_s32SM3BexvMaxPosIn/1 -> Before/13(sTmRefriVlvCtrl_X_s32SM3BexvMaxPosIn)
  yTmRefriVlvCtrl_B_EvapBattTLimBexvEnaIn/1 -> Before/14(yTmRefriVlvCtrl_B_EvapBattTLimBexvEnaIn)
  sTmRefriVlvCtrl_D_u8EexvRefriSwitchStIn/1 -> Before/15(sTmRefriVlvCtrl_D_u8EexvRefriSwitchStIn)
  sTmRefriVlvCtrl_D_u8CexvRefriSwitchStIn/1 -> Before/16(sTmRefriVlvCtrl_D_u8CexvRefriSwitchStIn)
  sTmRefriVlvCtrl_D_u8BexvRefriSwitchStIn/1 -> Before/17(sTmRefriVlvCtrl_D_u8BexvRefriSwitchStIn)
  Before/1(sTmRefriVlvCtrl_X_s32CEXVPosReq) -> sTmRefriVlvCtrl_X_s32CEXVPosReq/1
  Before/2(sTmRefriVlvCtrl_X_s32EEXVPosReq) -> sTmRefriVlvCtrl_X_s32EEXVPosReq/1
  Before/3(sTmRefriVlvCtrl_X_s32BEXVPosReq) -> sTmRefriVlvCtrl_X_s32BEXVPosReq/1
  Before/4(yTmRefriVlvCtrl_B_HpcCexvMovEnable) -> yTmRefriVlvCtrl_B_HpcCexvMovEnable/1
  Before/5(sTmRefriVlvCtrl_Z_u8CEXVInitState) -> sTmRefriVlvCtrl_Z_u8CEXVInitState/1
  Before/6(yTmRefriVlvCtrl_B_CexvCalibReq) -> yTmRefriVlvCtrl_B_CexvCalibReq/1
  Before/7(yTmRefriVlvCtrl_B_HpcEexvMovEnable) -> yTmRefriVlvCtrl_B_HpcEexvMovEnable/1
  Before/8(sTmRefriVlvCtrl_Z_u8EEXVInitState) -> sTmRefriVlvCtrl_Z_u8EEXVInitState/1
  Before/9(yTmRefriVlvCtrl_B_EexvCalibReq) -> yTmRefriVlvCtrl_B_EexvCalibReq/1
  Before/10(yTmRefriVlvCtrl_B_HpcBexvMovEnable) -> yTmRefriVlvCtrl_B_HpcBexvMovEnable/1
  Before/11(sTmRefriVlvCtrl_Z_u8BEXVInitState) -> sTmRefriVlvCtrl_Z_u8BEXVInitState/1
  Before/12(yTmRefriVlvCtrl_B_BexvCalibReq) -> yTmRefriVlvCtrl_B_BexvCalibReq/1
  Before/13(sTmRefriVlvCtrl_X_s32SM3BexvMaxPos) -> sTmRefriVlvCtrl_X_s32SM3BexvMaxPos/1
  Before/14(yTmRefriVlvCtrl_B_EvapBattTLimBexvEna) -> yTmRefriVlvCtrl_B_EvapBattTLimBexvEna/1
  Before/15(sTmRefriVlvCtrl_D_u8EexvRefriSwitchSt) -> sTmRefriVlvCtrl_D_u8EexvRefriSwitchSt/1
  Before/16(sTmRefriVlvCtrl_D_u8CexvRefriSwitchSt) -> sTmRefriVlvCtrl_D_u8CexvRefriSwitchSt/1
  Before/17(sTmRefriVlvCtrl_D_u8BexvRefriSwitchSt) -> sTmRefriVlvCtrl_D_u8BexvRefriSwitchSt/1

== system ScriptDemo/Create/createSigOnLine/Before1 ==
  sTmRefriVlvCtrl_X_s32CEXVPosReqIn : Inport  OutDataTypeStr=single  OutputFunctionCall=on
  sTmRefriVlvCtrl_X_s32EEXVPosReqIn : Inport  Port=2  OutDataTypeStr=single
  sTmRefriVlvCtrl_X_s32BEXVPosReqIn : Inport  Port=3  OutDataTypeStr=single
  yTmRefriVlvCtrl_B_HpcCexvMovEnableIn : Inport  Port=4  OutDataTypeStr=boolean
  sTmRefriVlvCtrl_Z_u8CEXVInitStateIn : Inport  Port=5  OutDataTypeStr=uint8
  yTmRefriVlvCtrl_B_CexvCalibReqIn : Inport  Port=6  OutDataTypeStr=boolean
  yTmRefriVlvCtrl_B_HpcEexvMovEnableIn : Inport  Port=7  OutDataTypeStr=boolean
  sTmRefriVlvCtrl_Z_u8EEXVInitStateIn : Inport  Port=8  OutDataTypeStr=uint8
  yTmRefriVlvCtrl_B_EexvCalibReqIn : Inport  Port=9  OutDataTypeStr=boolean
  yTmRefriVlvCtrl_B_HpcBexvMovEnableIn : Inport  Port=10  OutDataTypeStr=boolean
  sTmRefriVlvCtrl_Z_u8BEXVInitStateIn : Inport  Port=11  OutDataTypeStr=uint8
  yTmRefriVlvCtrl_B_BexvCalibReqIn : Inport  Port=12  OutDataTypeStr=boolean
  sTmRefriVlvCtrl_X_s32SM3BexvMaxPosIn : Inport  Port=13  OutDataTypeStr=single
  yTmRefriVlvCtrl_B_EvapBattTLimBexvEnaIn : Inport  Port=14  OutDataTypeStr=boolean
  sTmRefriVlvCtrl_D_u8EexvRefriSwitchStIn : Inport  Port=15  OutDataTypeStr=uint8
  sTmRefriVlvCtrl_D_u8CexvRefriSwitchStIn : Inport  Port=16  OutDataTypeStr=uint8
  sTmRefriVlvCtrl_D_u8BexvRefriSwitchStIn : Inport  Port=17  OutDataTypeStr=uint8
  Before : Subsystem
  sTmRefriVlvCtrl_X_s32CEXVPosReq : Outport  OutDataTypeStr=single
  sTmRefriVlvCtrl_X_s32EEXVPosReq : Outport  Port=2  OutDataTypeStr=single
  sTmRefriVlvCtrl_X_s32BEXVPosReq : Outport  Port=3  OutDataTypeStr=single
  yTmRefriVlvCtrl_B_HpcCexvMovEnable : Outport  Port=4  OutDataTypeStr=boolean
  sTmRefriVlvCtrl_Z_u8CEXVInitState : Outport  Port=5  OutDataTypeStr=uint8
  yTmRefriVlvCtrl_B_CexvCalibReq : Outport  Port=6  OutDataTypeStr=boolean
  yTmRefriVlvCtrl_B_HpcEexvMovEnable : Outport  Port=7  OutDataTypeStr=boolean
  sTmRefriVlvCtrl_Z_u8EEXVInitState : Outport  Port=8  OutDataTypeStr=uint8
  yTmRefriVlvCtrl_B_EexvCalibReq : Outport  Port=9  OutDataTypeStr=boolean
  yTmRefriVlvCtrl_B_HpcBexvMovEnable : Outport  Port=10  OutDataTypeStr=boolean
  sTmRefriVlvCtrl_Z_u8BEXVInitState : Outport  Port=11  OutDataTypeStr=uint8
  yTmRefriVlvCtrl_B_BexvCalibReq : Outport  Port=12  OutDataTypeStr=boolean
  sTmRefriVlvCtrl_X_s32SM3BexvMaxPos : Outport  Port=13  OutDataTypeStr=single
  yTmRefriVlvCtrl_B_EvapBattTLimBexvEna : Outport  Port=14  OutDataTypeStr=boolean
  sTmRefriVlvCtrl_D_u8EexvRefriSwitchSt : Outport  Port=15  OutDataTypeStr=uint8
  sTmRefriVlvCtrl_D_u8CexvRefriSwitchSt : Outport  Port=16  OutDataTypeStr=uint8
  sTmRefriVlvCtrl_D_u8BexvRefriSwitchSt : Outport  Port=17  OutDataTypeStr=uint8
  wires:
  sTmRefriVlvCtrl_X_s32CEXVPosReqIn/1 -> Before/1(sTmRefriVlvCtrl_X_s32CEXVPosReqIn)  "sTmRefriVlvCtrl_X_s32CEXVPosReqIn"
  sTmRefriVlvCtrl_X_s32EEXVPosReqIn/1 -> Before/2(sTmRefriVlvCtrl_X_s32EEXVPosReqIn)  "sTmRefriVlvCtrl_X_s32EEXVPosReqIn"
  sTmRefriVlvCtrl_X_s32BEXVPosReqIn/1 -> Before/3(sTmRefriVlvCtrl_X_s32BEXVPosReqIn)  "sTmRefriVlvCtrl_X_s32BEXVPosReqIn"
  yTmRefriVlvCtrl_B_HpcCexvMovEnableIn/1 -> Before/4(yTmRefriVlvCtrl_B_HpcCexvMovEnableIn)  "yTmRefriVlvCtrl_B_HpcCexvMovEnableIn"
  sTmRefriVlvCtrl_Z_u8CEXVInitStateIn/1 -> Before/5(sTmRefriVlvCtrl_Z_u8CEXVInitStateIn)  "sTmRefriVlvCtrl_Z_u8CEXVInitStateIn"
  yTmRefriVlvCtrl_B_CexvCalibReqIn/1 -> Before/6(yTmRefriVlvCtrl_B_CexvCalibReqIn)  "yTmRefriVlvCtrl_B_CexvCalibReqIn"
  yTmRefriVlvCtrl_B_HpcEexvMovEnableIn/1 -> Before/7(yTmRefriVlvCtrl_B_HpcEexvMovEnableIn)  "yTmRefriVlvCtrl_B_HpcEexvMovEnableIn"
  sTmRefriVlvCtrl_Z_u8EEXVInitStateIn/1 -> Before/8(sTmRefriVlvCtrl_Z_u8EEXVInitStateIn)  "sTmRefriVlvCtrl_Z_u8EEXVInitStateIn"
  yTmRefriVlvCtrl_B_EexvCalibReqIn/1 -> Before/9(yTmRefriVlvCtrl_B_EexvCalibReqIn)  "yTmRefriVlvCtrl_B_EexvCalibReqIn"
  yTmRefriVlvCtrl_B_HpcBexvMovEnableIn/1 -> Before/10(yTmRefriVlvCtrl_B_HpcBexvMovEnableIn)  "yTmRefriVlvCtrl_B_HpcBexvMovEnableIn"
  sTmRefriVlvCtrl_Z_u8BEXVInitStateIn/1 -> Before/11(sTmRefriVlvCtrl_Z_u8BEXVInitStateIn)  "sTmRefriVlvCtrl_Z_u8BEXVInitStateIn"
  yTmRefriVlvCtrl_B_BexvCalibReqIn/1 -> Before/12(yTmRefriVlvCtrl_B_BexvCalibReqIn)  "yTmRefriVlvCtrl_B_BexvCalibReqIn"
  sTmRefriVlvCtrl_X_s32SM3BexvMaxPosIn/1 -> Before/13(sTmRefriVlvCtrl_X_s32SM3BexvMaxPosIn)  "sTmRefriVlvCtrl_X_s32SM3BexvMaxPosIn"
  yTmRefriVlvCtrl_B_EvapBattTLimBexvEnaIn/1 -> Before/14(yTmRefriVlvCtrl_B_EvapBattTLimBexvEnaIn)  "yTmRefriVlvCtrl_B_EvapBattTLimBexvEnaIn"
  sTmRefriVlvCtrl_D_u8EexvRefriSwitchStIn/1 -> Before/15(sTmRefriVlvCtrl_D_u8EexvRefriSwitchStIn)  "sTmRefriVlvCtrl_D_u8EexvRefriSwitchStIn"
  sTmRefriVlvCtrl_D_u8CexvRefriSwitchStIn/1 -> Before/16(sTmRefriVlvCtrl_D_u8CexvRefriSwitchStIn)  "sTmRefriVlvCtrl_D_u8CexvRefriSwitchStIn"
  sTmRefriVlvCtrl_D_u8BexvRefriSwitchStIn/1 -> Before/17(sTmRefriVlvCtrl_D_u8BexvRefriSwitchStIn)  "sTmRefriVlvCtrl_D_u8BexvRefriSwitchStIn"
  Before/1(sTmRefriVlvCtrl_X_s32CEXVPosReq) -> sTmRefriVlvCtrl_X_s32CEXVPosReq/1  "sTmRefriVlvCtrl_X_s32CEXVPosReq"
  Before/2(sTmRefriVlvCtrl_X_s32EEXVPosReq) -> sTmRefriVlvCtrl_X_s32EEXVPosReq/1  "sTmRefriVlvCtrl_X_s32EEXVPosReq"
  Before/3(sTmRefriVlvCtrl_X_s32BEXVPosReq) -> sTmRefriVlvCtrl_X_s32BEXVPosReq/1  "sTmRefriVlvCtrl_X_s32BEXVPosReq"
  Before/4(yTmRefriVlvCtrl_B_HpcCexvMovEnable) -> yTmRefriVlvCtrl_B_HpcCexvMovEnable/1  "yTmRefriVlvCtrl_B_HpcCexvMovEnable"
  Before/5(sTmRefriVlvCtrl_Z_u8CEXVInitState) -> sTmRefriVlvCtrl_Z_u8CEXVInitState/1  "sTmRefriVlvCtrl_Z_u8CEXVInitState"
  Before/6(yTmRefriVlvCtrl_B_CexvCalibReq) -> yTmRefriVlvCtrl_B_CexvCalibReq/1  "yTmRefriVlvCtrl_B_CexvCalibReq"
  Before/7(yTmRefriVlvCtrl_B_HpcEexvMovEnable) -> yTmRefriVlvCtrl_B_HpcEexvMovEnable/1  "yTmRefriVlvCtrl_B_HpcEexvMovEnable"
  Before/8(sTmRefriVlvCtrl_Z_u8EEXVInitState) -> sTmRefriVlvCtrl_Z_u8EEXVInitState/1  "sTmRefriVlvCtrl_Z_u8EEXVInitState"
  Before/9(yTmRefriVlvCtrl_B_EexvCalibReq) -> yTmRefriVlvCtrl_B_EexvCalibReq/1  "yTmRefriVlvCtrl_B_EexvCalibReq"
  Before/10(yTmRefriVlvCtrl_B_HpcBexvMovEnable) -> yTmRefriVlvCtrl_B_HpcBexvMovEnable/1  "yTmRefriVlvCtrl_B_HpcBexvMovEnable"
  Before/11(sTmRefriVlvCtrl_Z_u8BEXVInitState) -> sTmRefriVlvCtrl_Z_u8BEXVInitState/1  "sTmRefriVlvCtrl_Z_u8BEXVInitState"
  Before/12(yTmRefriVlvCtrl_B_BexvCalibReq) -> yTmRefriVlvCtrl_B_BexvCalibReq/1  "yTmRefriVlvCtrl_B_BexvCalibReq"
  Before/13(sTmRefriVlvCtrl_X_s32SM3BexvMaxPos) -> sTmRefriVlvCtrl_X_s32SM3BexvMaxPos/1  "sTmRefriVlvCtrl_X_s32SM3BexvMaxPos"
  Before/14(yTmRefriVlvCtrl_B_EvapBattTLimBexvEna) -> yTmRefriVlvCtrl_B_EvapBattTLimBexvEna/1  "yTmRefriVlvCtrl_B_EvapBattTLimBexvEna"
  Before/15(sTmRefriVlvCtrl_D_u8EexvRefriSwitchSt) -> sTmRefriVlvCtrl_D_u8EexvRefriSwitchSt/1  "sTmRefriVlvCtrl_D_u8EexvRefriSwitchSt"
  Before/16(sTmRefriVlvCtrl_D_u8CexvRefriSwitchSt) -> sTmRefriVlvCtrl_D_u8CexvRefriSwitchSt/1  "sTmRefriVlvCtrl_D_u8CexvRefriSwitchSt"
  Before/17(sTmRefriVlvCtrl_D_u8BexvRefriSwitchSt) -> sTmRefriVlvCtrl_D_u8BexvRefriSwitchSt/1  "sTmRefriVlvCtrl_D_u8BexvRefriSwitchSt"

== system ScriptDemo/Create/createSigOnLine/Before2 ==
  sTmRefriVlvCtrl_X_s32CEXVPosReqIn : Inport  OutDataTypeStr=single  OutputFunctionCall=on
  sTmRefriVlvCtrl_X_s32EEXVPosReqIn : Inport  Port=2  OutDataTypeStr=single
  sTmRefriVlvCtrl_X_s32BEXVPosReqIn : Inport  Port=3  OutDataTypeStr=single
  yTmRefriVlvCtrl_B_HpcCexvMovEnableIn : Inport  Port=4  OutDataTypeStr=boolean
  sTmRefriVlvCtrl_Z_u8CEXVInitStateIn : Inport  Port=5  OutDataTypeStr=uint8
  yTmRefriVlvCtrl_B_CexvCalibReqIn : Inport  Port=6  OutDataTypeStr=boolean
  yTmRefriVlvCtrl_B_HpcEexvMovEnableIn : Inport  Port=7  OutDataTypeStr=boolean
  sTmRefriVlvCtrl_Z_u8EEXVInitStateIn : Inport  Port=8  OutDataTypeStr=uint8
  yTmRefriVlvCtrl_B_EexvCalibReqIn : Inport  Port=9  OutDataTypeStr=boolean
  yTmRefriVlvCtrl_B_HpcBexvMovEnableIn : Inport  Port=10  OutDataTypeStr=boolean
  sTmRefriVlvCtrl_Z_u8BEXVInitStateIn : Inport  Port=11  OutDataTypeStr=uint8
  yTmRefriVlvCtrl_B_BexvCalibReqIn : Inport  Port=12  OutDataTypeStr=boolean
  sTmRefriVlvCtrl_X_s32SM3BexvMaxPosIn : Inport  Port=13  OutDataTypeStr=single
  yTmRefriVlvCtrl_B_EvapBattTLimBexvEnaIn : Inport  Port=14  OutDataTypeStr=boolean
  sTmRefriVlvCtrl_D_u8EexvRefriSwitchStIn : Inport  Port=15  OutDataTypeStr=uint8
  sTmRefriVlvCtrl_D_u8CexvRefriSwitchStIn : Inport  Port=16  OutDataTypeStr=uint8
  sTmRefriVlvCtrl_D_u8BexvRefriSwitchStIn : Inport  Port=17  OutDataTypeStr=uint8
  Before : Subsystem
  sTmRefriVlvCtrl_X_s32CEXVPosReq : Outport  OutDataTypeStr=single
  sTmRefriVlvCtrl_X_s32EEXVPosReq : Outport  Port=2  OutDataTypeStr=single
  sTmRefriVlvCtrl_X_s32BEXVPosReq : Outport  Port=3  OutDataTypeStr=single
  yTmRefriVlvCtrl_B_HpcCexvMovEnable : Outport  Port=4  OutDataTypeStr=boolean
  sTmRefriVlvCtrl_Z_u8CEXVInitState : Outport  Port=5  OutDataTypeStr=uint8
  yTmRefriVlvCtrl_B_CexvCalibReq : Outport  Port=6  OutDataTypeStr=boolean
  yTmRefriVlvCtrl_B_HpcEexvMovEnable : Outport  Port=7  OutDataTypeStr=boolean
  sTmRefriVlvCtrl_Z_u8EEXVInitState : Outport  Port=8  OutDataTypeStr=uint8
  yTmRefriVlvCtrl_B_EexvCalibReq : Outport  Port=9  OutDataTypeStr=boolean
  yTmRefriVlvCtrl_B_HpcBexvMovEnable : Outport  Port=10  OutDataTypeStr=boolean
  sTmRefriVlvCtrl_Z_u8BEXVInitState : Outport  Port=11  OutDataTypeStr=uint8
  yTmRefriVlvCtrl_B_BexvCalibReq : Outport  Port=12  OutDataTypeStr=boolean
  sTmRefriVlvCtrl_X_s32SM3BexvMaxPos : Outport  Port=13  OutDataTypeStr=single
  yTmRefriVlvCtrl_B_EvapBattTLimBexvEna : Outport  Port=14  OutDataTypeStr=boolean
  sTmRefriVlvCtrl_D_u8EexvRefriSwitchSt : Outport  Port=15  OutDataTypeStr=uint8
  sTmRefriVlvCtrl_D_u8CexvRefriSwitchSt : Outport  Port=16  OutDataTypeStr=uint8
  sTmRefriVlvCtrl_D_u8BexvRefriSwitchSt : Outport  Port=17  OutDataTypeStr=uint8
  wires:
  sTmRefriVlvCtrl_X_s32CEXVPosReqIn/1 -> Before/1(sTmRefriVlvCtrl_X_s32CEXVPosReqIn)  "sTmRefriVlvCtrl_X_s32CEXVPosReqIn"
  sTmRefriVlvCtrl_X_s32EEXVPosReqIn/1 -> Before/2(sTmRefriVlvCtrl_X_s32EEXVPosReqIn)  "sTmRefriVlvCtrl_X_s32EEXVPosReqIn"
  sTmRefriVlvCtrl_X_s32BEXVPosReqIn/1 -> Before/3(sTmRefriVlvCtrl_X_s32BEXVPosReqIn)  "sTmRefriVlvCtrl_X_s32BEXVPosReqIn"
  yTmRefriVlvCtrl_B_HpcCexvMovEnableIn/1 -> Before/4(yTmRefriVlvCtrl_B_HpcCexvMovEnableIn)  "yTmRefriVlvCtrl_B_HpcCexvMovEnableIn"
  sTmRefriVlvCtrl_Z_u8CEXVInitStateIn/1 -> Before/5(sTmRefriVlvCtrl_Z_u8CEXVInitStateIn)  "sTmRefriVlvCtrl_Z_u8CEXVInitStateIn"
  yTmRefriVlvCtrl_B_CexvCalibReqIn/1 -> Before/6(yTmRefriVlvCtrl_B_CexvCalibReqIn)  "yTmRefriVlvCtrl_B_CexvCalibReqIn"
  yTmRefriVlvCtrl_B_HpcEexvMovEnableIn/1 -> Before/7(yTmRefriVlvCtrl_B_HpcEexvMovEnableIn)  "yTmRefriVlvCtrl_B_HpcEexvMovEnableIn"
  sTmRefriVlvCtrl_Z_u8EEXVInitStateIn/1 -> Before/8(sTmRefriVlvCtrl_Z_u8EEXVInitStateIn)  "sTmRefriVlvCtrl_Z_u8EEXVInitStateIn"
  yTmRefriVlvCtrl_B_EexvCalibReqIn/1 -> Before/9(yTmRefriVlvCtrl_B_EexvCalibReqIn)  "yTmRefriVlvCtrl_B_EexvCalibReqIn"
  yTmRefriVlvCtrl_B_HpcBexvMovEnableIn/1 -> Before/10(yTmRefriVlvCtrl_B_HpcBexvMovEnableIn)  "yTmRefriVlvCtrl_B_HpcBexvMovEnableIn"
  sTmRefriVlvCtrl_Z_u8BEXVInitStateIn/1 -> Before/11(sTmRefriVlvCtrl_Z_u8BEXVInitStateIn)  "sTmRefriVlvCtrl_Z_u8BEXVInitStateIn"
  yTmRefriVlvCtrl_B_BexvCalibReqIn/1 -> Before/12(yTmRefriVlvCtrl_B_BexvCalibReqIn)  "yTmRefriVlvCtrl_B_BexvCalibReqIn"
  sTmRefriVlvCtrl_X_s32SM3BexvMaxPosIn/1 -> Before/13(sTmRefriVlvCtrl_X_s32SM3BexvMaxPosIn)  "sTmRefriVlvCtrl_X_s32SM3BexvMaxPosIn"
  yTmRefriVlvCtrl_B_EvapBattTLimBexvEnaIn/1 -> Before/14(yTmRefriVlvCtrl_B_EvapBattTLimBexvEnaIn)  "yTmRefriVlvCtrl_B_EvapBattTLimBexvEnaIn"
  sTmRefriVlvCtrl_D_u8EexvRefriSwitchStIn/1 -> Before/15(sTmRefriVlvCtrl_D_u8EexvRefriSwitchStIn)  "sTmRefriVlvCtrl_D_u8EexvRefriSwitchStIn"
  sTmRefriVlvCtrl_D_u8CexvRefriSwitchStIn/1 -> Before/16(sTmRefriVlvCtrl_D_u8CexvRefriSwitchStIn)  "sTmRefriVlvCtrl_D_u8CexvRefriSwitchStIn"
  sTmRefriVlvCtrl_D_u8BexvRefriSwitchStIn/1 -> Before/17(sTmRefriVlvCtrl_D_u8BexvRefriSwitchStIn)  "sTmRefriVlvCtrl_D_u8BexvRefriSwitchStIn"
  Before/1(sTmRefriVlvCtrl_X_s32CEXVPosReq) -> sTmRefriVlvCtrl_X_s32CEXVPosReq/1  "sTmRefriVlvCtrl_X_s32CEXVPosReq"
  Before/2(sTmRefriVlvCtrl_X_s32EEXVPosReq) -> sTmRefriVlvCtrl_X_s32EEXVPosReq/1  "sTmRefriVlvCtrl_X_s32EEXVPosReq"
  Before/3(sTmRefriVlvCtrl_X_s32BEXVPosReq) -> sTmRefriVlvCtrl_X_s32BEXVPosReq/1  "sTmRefriVlvCtrl_X_s32BEXVPosReq"
  Before/4(yTmRefriVlvCtrl_B_HpcCexvMovEnable) -> yTmRefriVlvCtrl_B_HpcCexvMovEnable/1  "yTmRefriVlvCtrl_B_HpcCexvMovEnable"
  Before/5(sTmRefriVlvCtrl_Z_u8CEXVInitState) -> sTmRefriVlvCtrl_Z_u8CEXVInitState/1  "sTmRefriVlvCtrl_Z_u8CEXVInitState"
  Before/6(yTmRefriVlvCtrl_B_CexvCalibReq) -> yTmRefriVlvCtrl_B_CexvCalibReq/1  "yTmRefriVlvCtrl_B_CexvCalibReq"
  Before/7(yTmRefriVlvCtrl_B_HpcEexvMovEnable) -> yTmRefriVlvCtrl_B_HpcEexvMovEnable/1  "yTmRefriVlvCtrl_B_HpcEexvMovEnable"
  Before/8(sTmRefriVlvCtrl_Z_u8EEXVInitState) -> sTmRefriVlvCtrl_Z_u8EEXVInitState/1  "sTmRefriVlvCtrl_Z_u8EEXVInitState"
  Before/9(yTmRefriVlvCtrl_B_EexvCalibReq) -> yTmRefriVlvCtrl_B_EexvCalibReq/1  "yTmRefriVlvCtrl_B_EexvCalibReq"
  Before/10(yTmRefriVlvCtrl_B_HpcBexvMovEnable) -> yTmRefriVlvCtrl_B_HpcBexvMovEnable/1  "yTmRefriVlvCtrl_B_HpcBexvMovEnable"
  Before/11(sTmRefriVlvCtrl_Z_u8BEXVInitState) -> sTmRefriVlvCtrl_Z_u8BEXVInitState/1  "sTmRefriVlvCtrl_Z_u8BEXVInitState"
  Before/12(yTmRefriVlvCtrl_B_BexvCalibReq) -> yTmRefriVlvCtrl_B_BexvCalibReq/1  "yTmRefriVlvCtrl_B_BexvCalibReq"
  Before/13(sTmRefriVlvCtrl_X_s32SM3BexvMaxPos) -> sTmRefriVlvCtrl_X_s32SM3BexvMaxPos/1  "sTmRefriVlvCtrl_X_s32SM3BexvMaxPos"
  Before/14(yTmRefriVlvCtrl_B_EvapBattTLimBexvEna) -> yTmRefriVlvCtrl_B_EvapBattTLimBexvEna/1  "yTmRefriVlvCtrl_B_EvapBattTLimBexvEna"
  Before/15(sTmRefriVlvCtrl_D_u8EexvRefriSwitchSt) -> sTmRefriVlvCtrl_D_u8EexvRefriSwitchSt/1  "sTmRefriVlvCtrl_D_u8EexvRefriSwitchSt"
  Before/16(sTmRefriVlvCtrl_D_u8CexvRefriSwitchSt) -> sTmRefriVlvCtrl_D_u8CexvRefriSwitchSt/1  "sTmRefriVlvCtrl_D_u8CexvRefriSwitchSt"
  Before/17(sTmRefriVlvCtrl_D_u8BexvRefriSwitchSt) -> sTmRefriVlvCtrl_D_u8BexvRefriSwitchSt/1  "sTmRefriVlvCtrl_D_u8BexvRefriSwitchSt"
